simulink model "autopilot2e"  (R2020a)
settings: Solver=VariableStepAuto  StartTime=0.0  StopTime=250  RelTol=1e-3
values from neighbouring files (symbols this model uses):
  a = [-2.87]    [Assignment2e.m]    (also in task1d.m)
  aileron_limit = deg2rad(30)    [Assignment2e.m]    (also in task1d.m)
  b = [-0.65]    [Assignment2e.m]    (also in task1d.m)
  disturbance = deg2rad(1.5)    [Assignment2e.m]    (also in task1d.m)
  g = 9.81    [Assignment2e.m]    (also in task1d.m)
  kd_phi = (2*zeta_phi*omega_n_phi-a)/(b)    [Assignment2e.m]    (also in task1d.m)
  ki_phi = -0.15    [Assignment2e.m]    (also in task1d.m)
  ki_xi = omega_n_xi^2*Va/g    [Assignment2e.m]    (also in task1d.m)
  kp_phi = aileron_max/emax_phi*sign(b)    [Assignment2e.m]    (also in task1d.m)
  kp_xi = 2*zeta_xi*omega_n_xi*Va/g    [Assignment2e.m]    (also in task1d.m)
  Vg = Va    (= 580)    [Assignment2e.m]    (also in task1d.m)
settings Model: Creator=henab  LastModifiedBy=henab

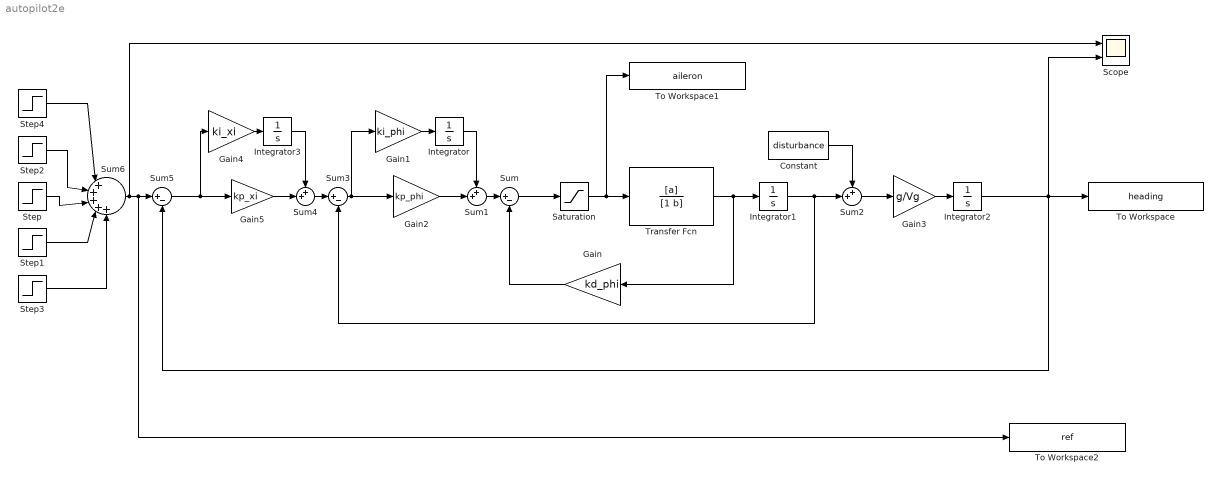
== system autopilot2e ==
  Constant : Constant  Value=disturbance
  Gain : Gain  Gain=kd_phi
  Gain1 : Gain  Gain=ki_phi
  Gain2 : Gain  Gain=kp_phi
  Gain3 : Gain  Gain=g/Vg
  Gain4 : Gain  Gain=ki_xi
  Gain5 : Gain  Gain=kp_xi
  Integrator{,1..3} (4 alike) : Integrator
  Saturation : Saturate  UpperLimit=aileron_limit  LowerLimit=-aileron_limit
  Scope : Scope  NumInputPorts=2
  Step : Step  Time=30  After=pi/12  SampleTime=0
  Step1 : Step  Time=50  After=-pi/24  SampleTime=0
  Step2 : Step  Time=150  After=0  SampleTime=0
  Step3 : Step  Time=180  After=pi/12  SampleTime=0
  Step4 : Step  Time=80  After=pi/12  SampleTime=0
  Sum : Sum  Inputs=|+-
  Sum1 : Sum  Inputs=++|
  Sum2 : Sum  Inputs=++|
  Sum3 : Sum  Inputs=|+-
  Sum4 : Sum  Inputs=++|
  Sum5 : Sum  Inputs=|+-
  Sum6 : Sum  Inputs=|+++++
  To Workspace : ToWorkspace  VariableName=heading  SaveFormat=Structure With Time  SampleTime=-1
  To Workspace1 : ToWorkspace  VariableName=aileron  SaveFormat=Structure With Time  SampleTime=-1
  To Workspace2 : ToWorkspace  VariableName=ref  SaveFormat=Structure With Time  SampleTime=-1
  Transfer Fcn : TransferFcn  Numerator=[a]  Denominator=[1 b]
  wires:
  Gain/1 -> Sum/2
  Gain1/1 -> Integrator/1
  Sum1/1 -> Sum/1
  Integrator/1 -> Sum1/1
  Gain2/1 -> Sum1/2
  Constant/1 -> Sum2/1
  Gain3/1 -> Integrator2/1
  Sum2/1 -> Gain3/1
  Integrator1/1 -> Sum2/2, Sum3/2
  Transfer Fcn/1 -> Gain/1, Integrator1/1
  Sum3/1 -> Gain1/1, Gain2/1
  Sum4/1 -> Sum3/1
  Gain4/1 -> Integrator3/1
  Integrator3/1 -> Sum4/1
  Gain5/1 -> Sum4/2
  Sum5/1 -> Gain4/1, Gain5/1
  Sum/1 -> Saturation/1
  Saturation/1 -> To Workspace1/1, Transfer Fcn/1
  Step4/1 -> Sum6/1
  Step2/1 -> Sum6/2
  Step/1 -> Sum6/3
  Step1/1 -> Sum6/4
  Step3/1 -> Sum6/5
  Sum6/1 -> Scope/1, To Workspace2/1, Sum5/1
  Integrator2/1 -> To Workspace/1, Scope/2, Sum5/2
